simulink model "HallEffect_Main"  (R2024a)
settings: Solver=VariableStepAuto  StartTime=0.0  StopTime=100  RelTol=1e-3
libraries: fl_lib x6, nesl_utility x4, spsEdgeDetectorLib x3, ee_lib x2, simulink_extras x1, dspswit3 x1
settings Model: Creator=lrada  LastModifiedBy=lrada

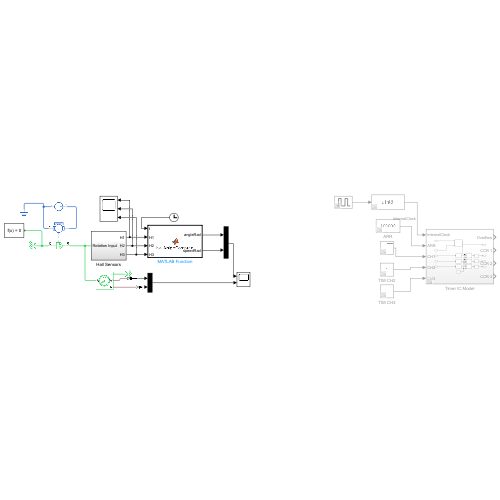
[thumbnail: Simulink's stored preview of the top-level diagram]
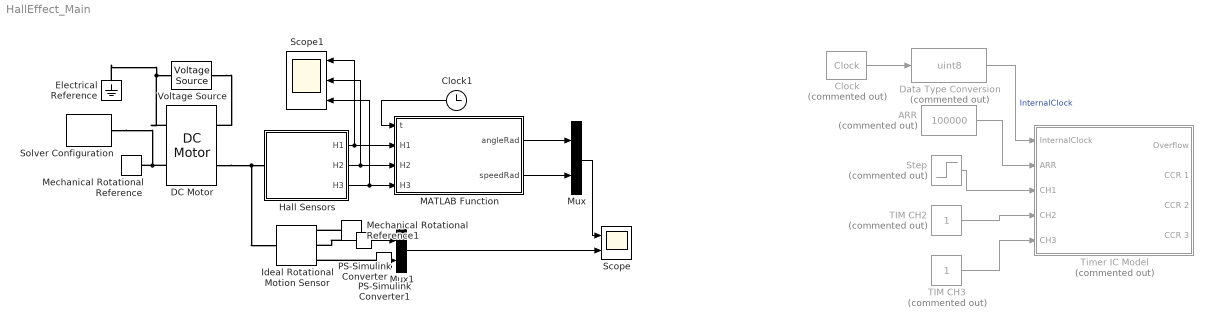
== system HallEffect_Main ==
  ARR : Constant  Commented=on  Value=100000  OutDataTypeStr=uint32
  Clock : simulink_extras/Flip Flops/Clock  Commented=on  period=1e-3
  Clock1 : Clock
  DC Motor : ee_lib/Electromechanical/Brushed Motors/DC Motor  field_option=ee.enum.field_option.pm  Rf=100 Ohm  Lf=1 H  Laf=0.15 H  If0=0 A  parameterization=ee.enum.dcparam_option.circuit_param  Ra=3.9 Ohm  La=12e-6 H  emf_or_torque=ee.enum.emf_or_torque.kv  Kv=0.01 V/rpm  Ki=6.876e-4 N*m/A  T_stall=0.24e-3 N*m  w_max=19100 rpm  w_rated=15000 rpm  P_rated=0.08 W  V_rated=1.5 V  lam_param=ee.enum.lam_param.damping  i_noload=0 A  V_i_noload=1.5 V  J=1 cm^2*g  lam=0 N*m*s/rad  speed0=0 rpm  enable_fault_armature=simscape.enum.onoff.off  rev_faulted=1 / 3  G_faulted_armature=1e-5 S  fault_trigger_armature=ee.enum.faults.faultTrigger.temporal  t_fault_armature=1 s  max_permissible_current_armature=inf A  t_fail_on_current_armature=1 s  enable_fault_field=simscape.enum.onoff.off  G_faulted_field=1e-5 S  fault_trigger_field=ee.enum.faults.faultTrigger.temporal  t_fault_field=1 s  max_permissible_current_field=inf A  t_fail_on_current_field=1 s  fault_action=simscape.enum.assert.action.none  alpha=3.93e-3 1/K  Tmeas=25 degC  thermal_mass=100 J/K  initial_temperature=25 degC
  Data Type Conversion : DataTypeConversion  Commented=on  OutDataTypeStr=uint8  SaturateOnIntegerOverflow=off  RndMeth=Floor
  Electrical Reference : fl_lib/Electrical/Electrical Elements/Electrical Reference
  Hall Sensors : Subsystem
  Ideal Rotational Motion Sensor : fl_lib/Mechanical/Mechanical Sensors/Ideal Rotational Motion Sensor  reference=foundation.enum.MeasurementReference.difference  acceleration_port=false  velocity_port=true  position_port=true  wrap_angle=false  offset=0 rad
  MATLAB Function : MATLAB Function  TreatAsAtomicUnit=on
  Mechanical Rotational Reference : fl_lib/Mechanical/Rotational Elements/Mechanical Rotational Reference
  Mechanical Rotational Reference1 : fl_lib/Mechanical/Rotational Elements/Mechanical Rotational Reference
  Mux : Mux  Inputs=2
  Mux1 : Mux  Inputs=2
  PS-Simulink Converter : nesl_utility/PS-Simulink Converter  PhysicalDomain=network_engine_domain  SubClassName=ps_output  LeftPortType=input  RightPortType=output  PseudoPeriodic=off  Frequencies=[]  VectorFormat=inherit  Unit=inherit  AffineConversion=off
  PS-Simulink Converter1 : nesl_utility/PS-Simulink Converter  PhysicalDomain=network_engine_domain  SubClassName=ps_output  LeftPortType=input  RightPortType=output  PseudoPeriodic=off  Frequencies=[]  VectorFormat=inherit  Unit=inherit  AffineConversion=off
  Scope : Scope  NumInputPorts=2
  Scope1 : Scope  NumInputPorts=3
  Solver Configuration : nesl_utility/Solver Configuration  PhysicalDomain=network_engine_domain  SubClassName=solver  LeftPortType=input  RightPortType=generic  Tones=[]  Harmonics=[]  SimulateNoise=off  Profile=off  UseLocalSampling=off  EnableSwitchedLinearOptims=on  FrequencyDomain=off  UseCCode=off  RelTol=0.001  AbsTol=0.001  MinStep=1e-09  ToWorkspace=off  RevertToSquareIcSolve=off  NumHomotopyIterations=100  PhasorMode=off  PhasorModeNumHarmonics=1  ConsistencySolver=NEWTON_XTOL_AFTER_FTOL  IndexReductionMethod=DerivativeReplacement  DoDC=off  ResidualTolerance=1e-09  ConsistencyTolSource=GLOBAL  ConsistencyAbsTol=0.001  ConsistencyRelTol=0.001  ConsistencyTolFactor=0.001  UseLocalSolver=off  LocalSolverChoice=NE_BACKWARD_EULER_ADVANCER  ResolveIndetEquations=on  FunctionEvalNumThread=1  LocalSolverSampleTime=0.001  DoFixedCost=off  MaxNonlinIter=3  MaxModeIter=2  ComputeImpulses=off  ImpulseIterations=2  LinearAlgebra=auto  LinearAlgebraNumThread=0  EquationFormulation=NE_TIME_EF  DelaysMemoryBudget=1024  AutomaticFiltering=on  FilteringTimeConstant=0.001  PartitionStorageMethod=AS_NEEDED  PartitionMemoryBudget=1024  PartitionMethod=ROBUST  MultibodyUseLocalSolver=off  MultibodyLocalSolverChoice=ODE1  MultibodyLocalSolverSampleTime=0.001
  Step : Step  Commented=on  Time=2  SampleTime=0
  TIM CH2 : Constant  Commented=on
  TIM CH3 : Constant  Commented=on
  Timer IC Model : Subsystem  Commented=on
  Voltage Source : ee_lib/Sources/Voltage Source  dc_voltage=5 V  ac_voltage=0 V  ac_shift=0 rad  ac_frequency=60 Hz  noise_mode=ee.enum.sources.noise.Disabled  PSD=0 V^2/Hz  sample_time=1e-3 s  repeatability=ee.enum.sources.repeatability.NotRepeatable  user_seed=0  auto_seed=3499211588  i_specify=off  i_priority=None  i=0 A  i_nominal_specify=off  i_nominal_value=1  i_nominal_unit=A  v_specify=off  v_priority=None  v=0 V  v_nominal_specify=off  v_nominal_value=1  v_nominal_unit=V
  wires:
  Clock/1 -> Data Type Conversion/1
  Data Type Conversion/1 -> Timer IC Model/1(InternalClock)  "InternalClock"
  ARR/1 -> Timer IC Model/2(ARR)
  TIM CH2/1 -> Timer IC Model/4(CH2)
  TIM CH3/1 -> Timer IC Model/5(CH3)
  Step/1 -> Timer IC Model/3(CH1)
  Hall Sensors/2(H2) -> Scope1/2, MATLAB Function/3(H2)
  Hall Sensors/1(H1) -> Scope1/1, MATLAB Function/2(H1)
  Clock1/1 -> MATLAB Function/1(t)
  MATLAB Function/1(angleRad) -> Mux/1
  MATLAB Function/2(speedRad) -> Mux/2
  Mux/1 -> Scope/1
  PS-Simulink Converter/1 -> Mux1/1
  PS-Simulink Converter1/1 -> Mux1/2
  Mux1/1 -> Scope/2
  Hall Sensors/3(H3) -> Scope1/3, MATLAB Function/4(H3)
  connections:
  Hall Sensors/LConn1 -- DC Motor/LConn2 -- Ideal Rotational Motion Sensor/LConn1
  DC Motor/RConn2 -- Solver Configuration/RConn1 -- Mechanical Rotational Reference/LConn1
  Mechanical Rotational Reference1/LConn1 -- Ideal Rotational Motion Sensor/RConn1
  PS-Simulink Converter/LConn1 -- Ideal Rotational Motion Sensor/RConn2
  PS-Simulink Converter1/LConn1 -- Ideal Rotational Motion Sensor/RConn3
  DC Motor/RConn1 -- Electrical Reference/LConn1 -- Voltage Source/RConn1
  Voltage Source/LConn1 -- DC Motor/LConn1

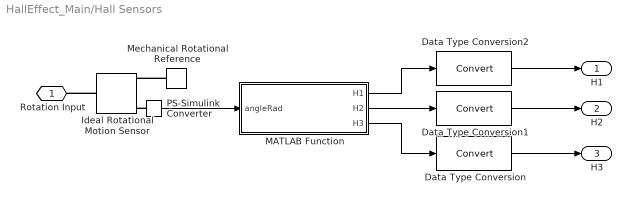
== system HallEffect_Main/Hall Sensors ==
  Data Type Conversion : DataTypeConversion  SaturateOnIntegerOverflow=off  RndMeth=Floor
  Data Type Conversion1 : DataTypeConversion  SaturateOnIntegerOverflow=off  RndMeth=Floor
  Data Type Conversion2 : DataTypeConversion  SaturateOnIntegerOverflow=off  RndMeth=Floor
  Ideal Rotational Motion Sensor : fl_lib/Mechanical/Mechanical Sensors/Ideal Rotational Motion Sensor  reference=foundation.enum.MeasurementReference.difference  acceleration_port=false  velocity_port=true  position_port=true  wrap_angle=false  offset=0 rad
  MATLAB Function : MATLAB Function  TreatAsAtomicUnit=on
  Mechanical Rotational Reference : fl_lib/Mechanical/Rotational Elements/Mechanical Rotational Reference
  PS-Simulink Converter : nesl_utility/PS-Simulink Converter  PhysicalDomain=network_engine_domain  SubClassName=ps_output  LeftPortType=input  RightPortType=output  PseudoPeriodic=off  Frequencies=[]  VectorFormat=inherit  Unit=inherit  AffineConversion=off
  Rotation Input : PMIOPort  Side=Left
  H1 : Outport  OutDataTypeStr=uint8
  H2 : Outport  Port=2  OutDataTypeStr=uint8
  H3 : Outport  Port=3  OutDataTypeStr=uint8
  wires:
  MATLAB Function/2(H2) -> Data Type Conversion1/1
  MATLAB Function/3(H3) -> Data Type Conversion/1
  PS-Simulink Converter/1 -> MATLAB Function/1(angleRad)
  MATLAB Function/1(H1) -> Data Type Conversion2/1
  Data Type Conversion/1 -> H3/1
  Data Type Conversion1/1 -> H2/1
  Data Type Conversion2/1 -> H1/1
  connections:
  PS-Simulink Converter/LConn1 -- Ideal Rotational Motion Sensor/RConn3
  Ideal Rotational Motion Sensor/LConn1 -- Rotation Input/RConn1
  Mechanical Rotational Reference/LConn1 -- Ideal Rotational Motion Sensor/RConn1

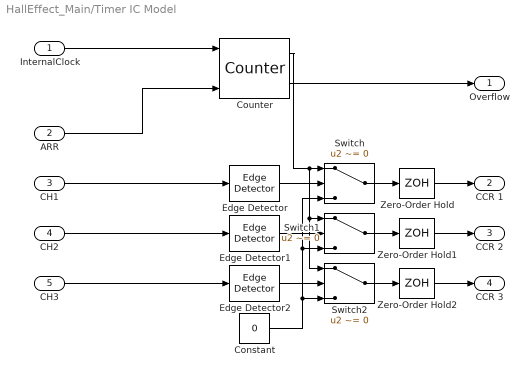
== system HallEffect_Main/Timer IC Model ==
  InternalClock : Inport
  ARR : Inport  Port=2
  CH1 : Inport  Port=3
  CH2 : Inport  Port=4
  CH3 : Inport  Port=5
  Constant : Constant  Value=0
  Counter : dspswit3/Counter  Direction=Up  CountEvent=Rising edge  CounterSize=Specify via input port  MaxCount=255  InitialCount=0  Output=Count and Hit  HitValue=32  ResetInput=on  SamplesPerFrame=1  Ts=1  CntDtype=double  HitDtype=Logical
  Edge Detector : spsEdgeDetectorLib/Edge Detector  model=Rising  ic=0  Ts=0
      settings: LibrarySourceBlock=sps_lib/Control/Edge Detector
  Edge Detector1 : spsEdgeDetectorLib/Edge Detector  model=Rising  ic=0  Ts=0
      settings: LibrarySourceBlock=sps_lib/Control/Edge Detector
  Edge Detector2 : spsEdgeDetectorLib/Edge Detector  model=Rising  ic=0  Ts=0
      settings: LibrarySourceBlock=sps_lib/Control/Edge Detector
  Switch : Switch  Criteria=u2 ~= 0  SaturateOnIntegerOverflow=off  InputSameDT=off
  Switch1 : Switch  Criteria=u2 ~= 0  SaturateOnIntegerOverflow=off  InputSameDT=off
  Switch2 : Switch  Criteria=u2 ~= 0  SaturateOnIntegerOverflow=off  InputSameDT=off
  Zero-Order Hold : ZeroOrderHold  SampleTime=-1
  Zero-Order Hold1 : ZeroOrderHold  SampleTime=-1
  Zero-Order Hold2 : ZeroOrderHold  SampleTime=-1
  Overflow : Outport
  CCR 1 : Outport  Port=2
  CCR 2 : Outport  Port=3
  CCR 3 : Outport  Port=4
  wires:
  Edge Detector2/1 -> Switch2/2
  Zero-Order Hold/1 -> CCR 1/1
  InternalClock/1 -> Counter/1
  Zero-Order Hold1/1 -> CCR 2/1
  Switch1/1 -> Zero-Order Hold1/1
  Switch/1 -> Zero-Order Hold/1
  ARR/1 -> Counter/3
  Zero-Order Hold2/1 -> CCR 3/1
  Counter/2 -> Overflow/1
  Edge Detector/1 -> Switch/2
  Counter/1 -> Switch1/1, Switch2/1, Switch/1
  Edge Detector1/1 -> Switch1/2
  Switch2/1 -> Zero-Order Hold2/1
  CH1/1 -> Edge Detector/1
  CH3/1 -> Edge Detector2/1
  CH2/1 -> Edge Detector1/1
  Constant/1 -> Switch/3, Switch1/3, Switch2/3

== matlab function HallEffect_Main/MATLAB Function ==
  settings: updateMethod=DISCRETE  sampleTime=1e-3
  data: t input double; H1 input uint8; H2 input uint8; H3 input uint8; angleRad output; speedRad output
function [angleRad, speedRad] = hallAnlgeCompute(t, H1, H2, H3)

    % HALL_OUT_LUT_60 = [1,0,1;1,0,0;1,1,0;0,1,0;0,1,1;0,0,1];
    persistent internalSpeed
    persistent oldAngle
    persistent oldTime

    if isempty(internalSpeed)
        internalSpeed = 0;
    end
    if isempty(oldAngle)
        oldAngle = (0);
    end
    if isempty(oldTime)
        oldTime = (0);
    end
    
    
    hallReading = bitor(bitshift(H2, 1), bitshift(H3, 2));
    hallReading = bitor(hallReading, bitshift(H1, 0));

    angleApprox = 0;
    switch hallReading
        case 0b101
            angleApprox = 0;
        case 0b100
            angleApprox = 60;
        case 0b110
            angleApprox = 120;
        case 0b010
            angleApprox = 180;
        case 0b011
            angleApprox = 240;
        case 0b001
            angleApprox = 300;
    end
    
    if angleApprox ~= oldAngle
        deltaT = t - oldTime;
        % deltaAngle = oldAngle - angleApprox; % Adjust direction here
        deltaAngle = 60;
        speedDeg = deltaAngle / deltaT;
        internalSpeed = speedDeg * (pi/180);
        oldAngle = angleApprox;
        oldTime = t;
    end

    angleRad = oldAngle + (t-oldTime) * internalSpeed;
    speedRad = internalSpeed;

    
end

== matlab function HallEffect_Main/Hall Sensors/MATLAB Function ==
  settings: updateMethod=DISCRETE  sampleTime=1e-3
  data: angleRad input; H1 output; H2 output; H3 output
function [H1, H2, H3] = angle2hall(angleRad)

HALL_DEGREES = 60;

% The LUT was built according to maxon catalogue page 67
% https://online.flippingbook.com/view/398826/67/#zoom=true

HALL_OUT_LUT_60 = [1,0,1;1,0,0;1,1,0;0,1,0;0,1,1;0,0,1];

angleDeg = angleRad * (180/pi);

anglePosition = round(angleDeg/HALL_DEGREES) + 1;
if anglePosition > 6
    anglePosition = 1;
end

H1 = HALL_OUT_LUT_60(anglePosition,1);
H2 = HALL_OUT_LUT_60(anglePosition,2);
H3 = HALL_OUT_LUT_60(anglePosition,3);




end
